simulink model "lqi8_discreto"  (R2025b)
settings: Solver=VariableStepAuto  StartTime=0.0  StopTime=10  RelTol=1e-3
undefined symbols (not defined in the file or in its folder): C, dK, dL, dsys
settings Model: Creator=rel  LastModifiedBy=rel

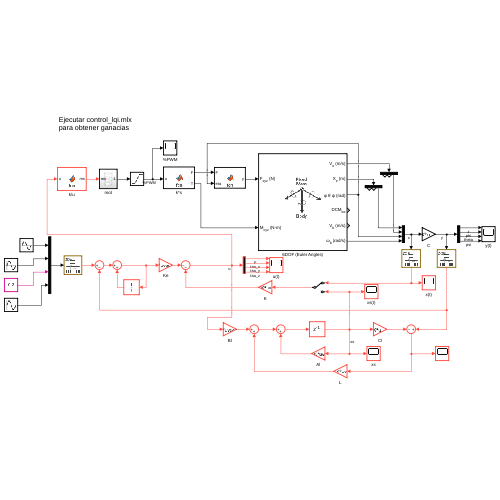
[thumbnail: Simulink's stored preview of the top-level diagram]
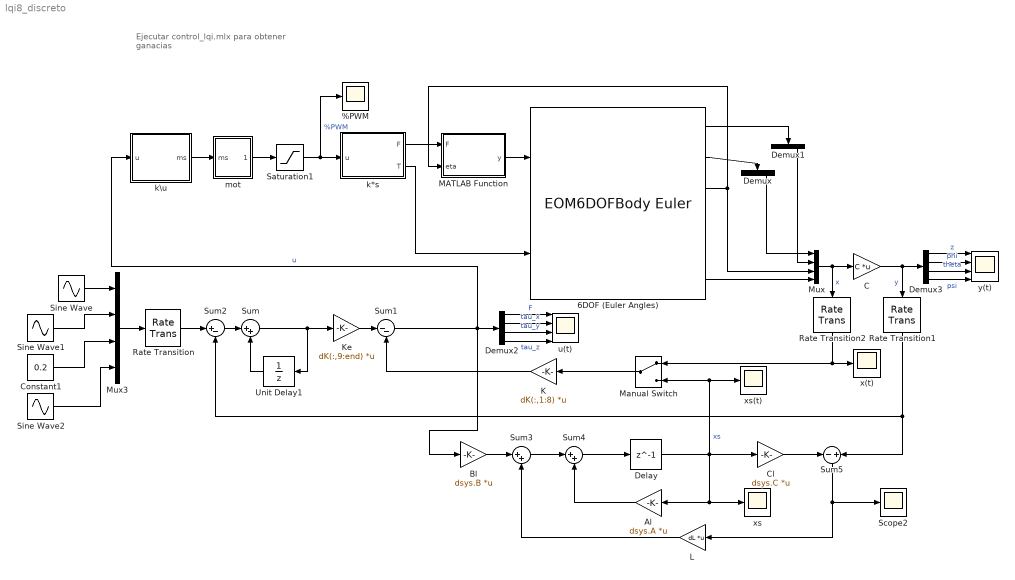
== system lqi8_discreto ==
  note: Ejecutar control_lqi.mlx
      | para obtener ganacias
  %PWM : Scope
      settings: ActiveDisplayYMinimum=-0.11019997872952345  ActiveDisplayYMaximum=0.99179980856571126  DataLoggingVariableName=ScopeData4
  6DOF (Euler Angles) : EOM6DOFBodyEuler  mass_0=1.6  inertia=diag([0.021915027 0.022124548 0.042349865])
  Al : Gain  Gain=dsys.A  Multiplication=Matrix(K*u) (u vector)
  Bl : Gain  Gain=dsys.B  Multiplication=Matrix(K*u) (u vector)
  C : Gain  Gain=C  Multiplication=Matrix(K*u)
  Cl : Gain  Gain=dsys.C  Multiplication=Matrix(K*u)
  Constant1 : Constant  Value=0.2
  Delay : Delay  DelayLength=1
  Demux : Demux  Outputs=3
  Demux1 : Demux  Outputs=3
  Demux2 : Demux
  Demux3 : Demux
  K : Gain  Gain=dK(:,1:8)  Multiplication=Matrix(K*u) (u vector)
  Ke : Gain  Gain=dK(:,9:end)  Multiplication=Matrix(K*u) (u vector)
  L : Gain  Gain=dL  Multiplication=Matrix(K*u) (u vector)
  MATLAB Function : MATLAB Function  TreatAsAtomicUnit=on
  Manual Switch : ManualSwitch
  Mux : Mux
  Mux3 : Mux
  Rate Transition : RateTransition  OutPortSampleTime=1/510
  Rate Transition1 : RateTransition  OutPortSampleTime=1/510
  Rate Transition2 : RateTransition  OutPortSampleTime=1/510
  Saturation1 : Saturate  UpperLimit=1  LowerLimit=0
  Scope2 : Scope
      settings: ActiveDisplayYMinimum=-7.4254678983131941E+307  ActiveDisplayYMaximum=3.2718910055311481E+307  DataLoggingVariableName=ScopeData6
  Sine Wave : Sin  Amplitude=0.5  Bias=1  Frequency=2  SampleTime=0
  Sine Wave1 : Sin  Amplitude=0.3  Frequency=3  SampleTime=0
  Sine Wave2 : Sin  SampleTime=0
  Sum : Sum  Inputs=|++
  Sum1 : Sum  Inputs=|--
  Sum2 : Sum  Inputs=|+-
  Sum3 : Sum  Inputs=|++
  Sum4 : Sum  Inputs=|++
  Sum5 : Sum  Inputs=-|+
  Unit Delay1 : UnitDelay  SampleTime=1/510  HasFrameUpgradeWarning=on
  k*s : MATLAB Function  TreatAsAtomicUnit=on
  k\u : MATLAB Function  TreatAsAtomicUnit=on
  mot : Subsystem
  u(t) : Scope  NumInputPorts=4
      settings: ActiveDisplayYMinimum=-2.8297706098234969  ActiveDisplayYMaximum=26.458782486419803
  x(t) : Scope
      settings: ActiveDisplayYMinimum=-1.2667564851369479  ActiveDisplayYMaximum=1.8612667832964724  DataLoggingVariableName=ScopeData3
  xs : Scope
      settings: ActiveDisplayYMinimum=-7.6172906269775348E+307  ActiveDisplayYMaximum=1.4297720503395759E+308  DataLoggingVariableName=ScopeData5
  xs(t) : Scope
      settings: ActiveDisplayYMinimum=-1.1261241911523992E+308  ActiveDisplayYMaximum=8.3131735545346209E+307  DataLoggingVariableName=ScopeData7
  y(t) : Scope  NumInputPorts=4
      settings: ActiveDisplayYMinimum=-0.30939395848760343  ActiveDisplayYMaximum=1.5827748939924511
  wires:
  C/1 -> Demux3/1, Rate Transition1/1  "y"
  K/1 -> Sum1/2
  Sum/1 -> Ke/1, Unit Delay1/1
  6DOF (Euler Angles)/2 -> Demux/1
  6DOF (Euler Angles)/3 -> Mux/3, MATLAB Function/2(eta)
  6DOF (Euler Angles)/1 -> Demux1/1
  mot/1(Out1) -> Saturation1/1
  k\u/1(ms) -> mot/1(ms)
  Saturation1/1 -> %PWM/1, k*s/1(u)  "%PWM"
  k*s/2(T) -> 6DOF (Euler Angles)/2
  Sine Wave/1 -> Mux3/1
  k*s/1(F) -> MATLAB Function/1(F)
  MATLAB Function/1(y) -> 6DOF (Euler Angles)/1
  Bl/1 -> Sum3/1
  Sum3/1 -> Sum4/1
  Delay/1 -> Al/1, xs/1, Manual Switch/2, xs(t)/1, Cl/1  "xs"
  Cl/1 -> Sum5/1
  Al/1 -> Sum4/2
  L/1 -> Sum3/2
  Sum5/1 -> L/1, Scope2/1
  Demux/3 -> Mux/1
  Demux1/3 -> Mux/2
  6DOF (Euler Angles)/6 -> Mux/4
  Mux/1 -> Rate Transition2/1, C/1  "x"
  Manual Switch/1 -> K/1
  Sum4/1 -> Delay/1
  Unit Delay1/1 -> Sum/2
  Sum2/1 -> Sum/1
  Ke/1 -> Sum1/1
  Mux3/1 -> Rate Transition/1
  Sum1/1 -> Demux2/1, Bl/1, k\u/1(u)  "u"
  Sine Wave1/1 -> Mux3/2
  Constant1/1 -> Mux3/3
  Sine Wave2/1 -> Mux3/4
  Demux2/1 -> u(t)/1  "F"
  Demux2/2 -> u(t)/2  "tau_x"
  Demux2/3 -> u(t)/3  "tau_y"
  Demux2/4 -> u(t)/4  "tau_z"
  Demux3/1 -> y(t)/1  "z"
  Demux3/2 -> y(t)/2  "phi"
  Demux3/3 -> y(t)/3  "theta"
  Demux3/4 -> y(t)/4  "psi"
  Rate Transition/1 -> Sum2/1
  Rate Transition1/1 -> Sum2/2, Sum5/2
  Rate Transition2/1 -> Manual Switch/1, x(t)/1

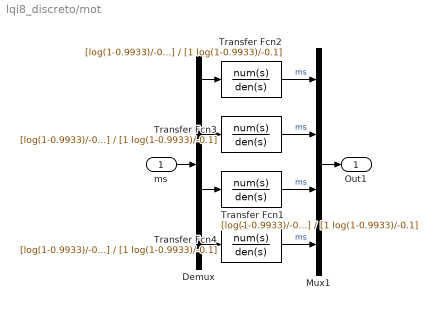
== system lqi8_discreto/mot ==
  ms : Inport
  Demux : Demux
  Mux1 : Mux
  Transfer Fcn{1..4} (4 alike) : TransferFcn  Numerator=[log(1-0.9933)/-0.1]  Denominator=[1 log(1-0.9933)/-0.1]
  Out1 : Outport
  wires:
  Transfer Fcn3/1 -> Mux1/2  "ms"
  Transfer Fcn1/1 -> Mux1/3  "ms"
  Demux/3 -> Transfer Fcn1/1
  Transfer Fcn4/1 -> Mux1/4  "ms"
  Demux/4 -> Transfer Fcn4/1
  Mux1/1 -> Out1/1
  Transfer Fcn2/1 -> Mux1/1  "ms"
  Demux/2 -> Transfer Fcn3/1
  Demux/1 -> Transfer Fcn2/1
  ms/1 -> Demux/1

== matlab function lqi8_discreto/k\u ==
  data: u input; ms output
function ms = fcn(u)
% L = 0.0080;
% kF = 0.1600*9.81;
% kM = 0.0086;
L = 0.268554;
kF = 7.965;
kM = 0.2;
A = [kF kF kF kF; -L*kF -L*kF L*kF L*kF; L*kF -L*kF -L*kF L*kF; -kM kM -kM kM];
ms = A\[u(1); u(2:end)];

== matlab function lqi8_discreto/MATLAB Function ==
  data: F input; y output; eta input
function y = fcn(F, eta)
phi = eta(1);
theta = eta(2);
psi = eta(3);
y = [0;0;-1.6*9.81] + [sin(theta)*cos(psi) + sin(phi)*cos(theta)*sin(psi); ...
                    sin(theta)*sin(psi) - sin(phi)*cos(theta)*cos(psi); ...
                    cos(phi)*cos(theta)]*F;

== matlab function lqi8_discreto/k*s ==
  data: u input; F output; T output
function [F, T] = fcn(u)
% L = 0.0080;
% kF = 0.1600*9.81;
% kM = 0.0086;
L = 0.268554;
kF = 7.965;
kM = 0.2;
A = [kF kF kF kF; -L*kF -L*kF L*kF L*kF; L*kF -L*kF -L*kF L*kF; -kM kM -kM kM];
y = A*u;
F = y(1);
T = y(2:end);
